simulink model "sigm"  (R2015a)
settings: Solver=ode45  StartTime=0.0  StopTime=20.0  RelTol=1e-3
values from neighbouring files (symbols this model uses):
  YG = 0.8    [NNPID.m]
libraries: simulink x1
settings Model: Creator=ANSYSVLAD  LastModifiedBy=ANSYSVLAD

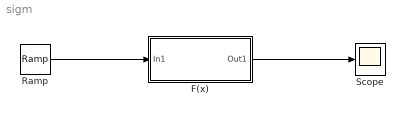
== system sigm ==
  F(x) : Subsystem
  Ramp : simulink/Sources/Ramp  slope=1  start=0  X0=-10
  Scope : Scope
  wires:
  F(x)/1(Out1) -> Scope/1
  Ramp/1 -> F(x)/1(In1)

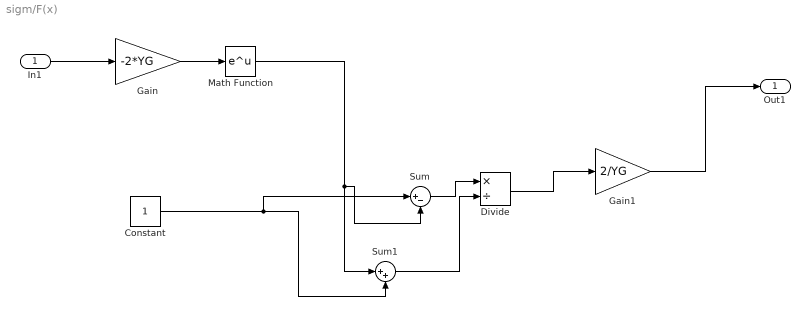
== system sigm/F(x) ==
  In1 : Inport
  Constant : Constant
  Divide : Product  Inputs=*/
  Gain : Gain  Gain=-2*YG
  Gain1 : Gain  Gain=2/YG
  Math Function : Math  SaturateOnIntegerOverflow=on
  Sum : Sum  Inputs=|+-
  Sum1 : Sum  Inputs=|++
  Out1 : Outport
  wires:
  In1/1 -> Gain/1
  Gain/1 -> Math Function/1
  Constant/1 -> Sum1/2, Sum/1
  Math Function/1 -> Sum1/1, Sum/2
  Sum/1 -> Divide/1
  Sum1/1 -> Divide/2
  Divide/1 -> Gain1/1
  Gain1/1 -> Out1/1
